simulink model "ejh61a"  (Simulink 3.00)
settings: Solver=ode45  StartTime=0.0  StopTime=10.0  RelTol=1e-3
values from neighbouring files (symbols this model uses):
  x = P_global(1,:)'    [contp5.m]    (also in ejh31.m = [0:0.2:5]; ejh62.m = 0:0.01:12; ejh63.m = 0:0.01:12)
  y = P_global(2,:)'    [contp5.m]    (also in ejh31.m = sqrt(25-x.^2); ejh62.m = 0:0.01:12; ejh63.m = 0:0.01:12)
undefined symbols (not defined in the file or in its folder): L
settings Model: LastModifiedBy=Administrador

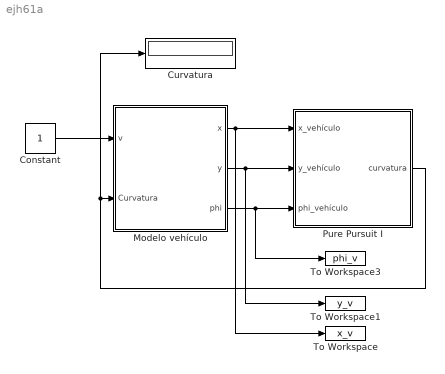
== system ejh61a ==
  Constant : Constant  Value=1
  Curvatura : Display
      settings: Format=short
  Modelo vehículo : Subsystem  mask{x_inicial=0, y_inicial=0.5, phi_inicial=0}
      mask prompts: x_inicial "Valor inicial de la coordenada x:"; y_inicial "Valor inicial de la coordenada y:"; phi_inicial "Valor inicial de la orientación:"
  Pure Pursuit I : Subsystem  mask(Pure Pursuit I){x_camino=x, y_camino=y, L=L}
      mask prompts: x_camino "Coordenadas x del camino:"; y_camino "Coordenadas y del camino:"; L "Parámetro Look-ahead (L):"
      mask help: Este bloque se encarga de calcular la curvatura que es necesario suministrar al vehículo cuando se emplea la técnica de persecución pura con el parámetro look-ahead (L) fijo.
      mask init:
      | global K_ANT
      | K_ANT=1;
  To Workspace : ToWorkspace  VariableName=x_v  SampleTime=-1  SaveFormat=Matrix
  To Workspace1 : ToWorkspace  VariableName=y_v  SampleTime=-1  SaveFormat=Matrix
  To Workspace3 : ToWorkspace  VariableName=phi_v  SampleTime=-1  SaveFormat=Matrix
  wires:
  Constant/1 -> Modelo vehículo/1(v)
  Modelo vehículo/1(x) -> To Workspace/1, Pure Pursuit I/1(x_vehículo)
  Pure Pursuit I/1(curvatura) -> Modelo vehículo/2(Curvatura), Curvatura/1
  Modelo vehículo/2(y) -> To Workspace1/1, Pure Pursuit I/2(y_vehículo)
  Modelo vehículo/3(phi) -> Pure Pursuit I/3(phi_vehículo), To Workspace3/1

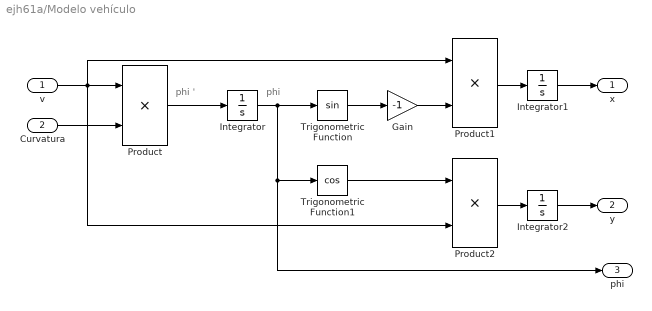
== system ejh61a/Modelo vehículo ==
  note: phi '
  note: phi
  v : Inport  Port=1  PortWidth=-1  SampleTime=-1  DataType=auto
      settings: SignalType=auto
  Curvatura : Inport  Port=2  PortWidth=-1  SampleTime=-1  DataType=auto
      settings: SignalType=auto
  Gain : Gain  Gain=-1  SaturateOnIntegerOverflow=on
  Integrator : Integrator  ExternalReset=none  InitialConditionSource=internal  InitialCondition=phi_inicial  LimitOutput=off  UpperSaturationLimit=inf  LowerSaturationLimit=-inf  ShowSaturationPort=off  ShowStatePort=off  AbsoluteTolerance=auto
  Integrator1 : Integrator  ExternalReset=none  InitialConditionSource=internal  InitialCondition=x_inicial  LimitOutput=off  UpperSaturationLimit=inf  LowerSaturationLimit=-inf  ShowSaturationPort=off  ShowStatePort=off  AbsoluteTolerance=auto
  Integrator2 : Integrator  ExternalReset=none  InitialConditionSource=internal  InitialCondition=y_inicial  LimitOutput=off  UpperSaturationLimit=inf  LowerSaturationLimit=-inf  ShowSaturationPort=off  ShowStatePort=off  AbsoluteTolerance=auto
  Product : Product  Inputs=2  SaturateOnIntegerOverflow=on
  Product1 : Product  Inputs=2  SaturateOnIntegerOverflow=on
  Product2 : Product  Inputs=2  SaturateOnIntegerOverflow=on
  Trigonometric Function : Trigonometry  Operator=sin  OutputSignalType=auto
  Trigonometric Function1 : Trigonometry  Operator=cos  OutputSignalType=auto
  x : Outport  Port=1
  y : Outport  Port=2
  phi : Outport  Port=3
  wires:
  Curvatura/1 -> Product/2
  Product/1 -> Integrator/1
  Integrator/1 -> Trigonometric Function/1, Trigonometric Function1/1, phi/1
  Trigonometric Function/1 -> Gain/1
  Gain/1 -> Product1/2
  v/1 -> Product/1, Product1/1, Product2/2
  Trigonometric Function1/1 -> Product2/1
  Product1/1 -> Integrator1/1
  Product2/1 -> Integrator2/1
  Integrator2/1 -> y/1
  Integrator1/1 -> x/1

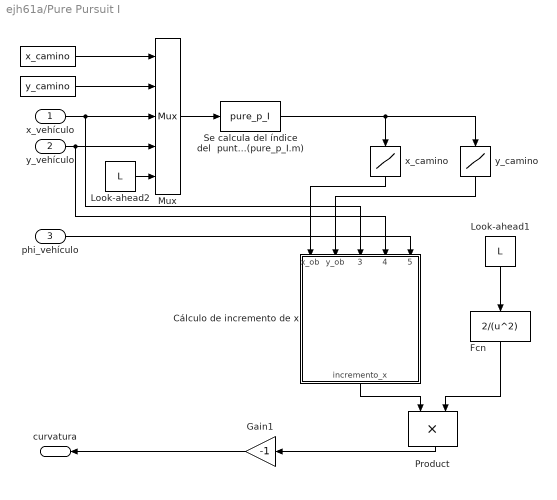
== system ejh61a/Pure Pursuit I ==
  x_vehículo : Inport  Port=1  PortWidth=-1  SampleTime=-1  DataType=auto
      settings: SignalType=auto
  y_vehículo : Inport  Port=2  PortWidth=-1  SampleTime=-1  DataType=auto
      settings: SignalType=auto
  phi_vehículo : Inport  Port=3  PortWidth=-1  SampleTime=-1  DataType=auto
      settings: SignalType=auto
  " " : Constant  Value=y_camino
  "  " : Constant  Value=x_camino
  Cálculo de incremento de x : Subsystem  Orientation=down
  Fcn : Fcn  Orientation=down  Expr=2/(u^2)
  Gain1 : Gain  Orientation=left  Gain=-1  SaturateOnIntegerOverflow=on
  Look-ahead1 : Constant  Orientation=down  Value=L
  Look-ahead2 : Constant  Value=L
  Mux : Mux  Inputs=5
      settings: DisplayOption=none
  Product : Product  Orientation=down  Inputs=2  SaturateOnIntegerOverflow=on
  Se calcula del índice del  punto que está a distancia L (pure_p_I.m) : MATLABFcn  MATLABFcn=pure_p_I  OutputWidth=-1  OutputSignalType=auto
  x_camino : Lookup  Orientation=down  InputValues=1:length(x_camino)  OutputValues=x_camino
  y_camino : Lookup  Orientation=down  InputValues=1:length(y_camino)  OutputValues=y_camino
  curvatura : Outport  Orientation=left  Port=1
  wires:
  Fcn/1 -> Product/2
  Look-ahead1/1 -> Fcn/1
  Se calcula del índice del  punto que está a distancia L (pure_p_I.m)/1 -> y_camino/1, x_camino/1
  y_camino/1 -> Cálculo de incremento de x/2(y_ob)
  x_camino/1 -> Cálculo de incremento de x/1(x_ob)
  Gain1/1 -> curvatura/1
  Product/1 -> Gain1/1
  "  "/1 -> Mux/1
  " "/1 -> Mux/2
  x_vehículo/1 -> Mux/3, Cálculo de incremento de x/3(x_vehículo)
  y_vehículo/1 -> Mux/4, Cálculo de incremento de x/4(y_vehículo)
  Look-ahead2/1 -> Mux/5
  Mux/1 -> Se calcula del índice del  punto que está a distancia L (pure_p_I.m)/1
  Cálculo de incremento de x/1(incremento_x) -> Product/1
  phi_vehículo/1 -> Cálculo de incremento de x/5(phi_vehículo)

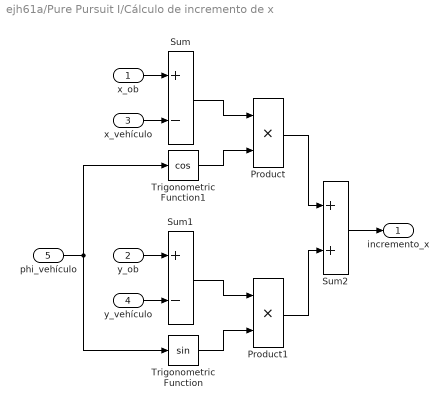
== system ejh61a/Pure Pursuit I/Cálculo de incremento de x ==
  x_ob : Inport  Port=1  PortWidth=-1  SampleTime=-1  DataType=auto
      settings: SignalType=auto
  y_ob : Inport  Port=2  PortWidth=-1  SampleTime=-1  DataType=auto
      settings: SignalType=auto
  x_vehículo : Inport  Port=3  PortWidth=-1  SampleTime=-1  DataType=auto
      settings: SignalType=auto
  y_vehículo : Inport  Port=4  PortWidth=-1  SampleTime=-1  DataType=auto
      settings: SignalType=auto
  phi_vehículo : Inport  Port=5  PortWidth=-1  SampleTime=-1  DataType=auto
      settings: SignalType=auto
  Product : Product  Inputs=2  SaturateOnIntegerOverflow=on
  Product1 : Product  Inputs=2  SaturateOnIntegerOverflow=on
  Sum : Sum  Inputs=+-  SaturateOnIntegerOverflow=on
  Sum1 : Sum  Inputs=+-  SaturateOnIntegerOverflow=on
  Sum2 : Sum  Inputs=++  SaturateOnIntegerOverflow=on
  Trigonometric Function : Trigonometry  Operator=sin  OutputSignalType=auto
  Trigonometric Function1 : Trigonometry  Operator=cos  OutputSignalType=auto
  incremento_x : Outport  Port=1
  wires:
  Sum2/1 -> incremento_x/1
  Product1/1 -> Sum2/2
  Product/1 -> Sum2/1
  Trigonometric Function/1 -> Product1/2
  Sum1/1 -> Product1/1
  phi_vehículo/1 -> Trigonometric Function/1, Trigonometric Function1/1
  Trigonometric Function1/1 -> Product/2
  Sum/1 -> Product/1
  y_vehículo/1 -> Sum1/2
  y_ob/1 -> Sum1/1
  x_vehículo/1 -> Sum/2
  x_ob/1 -> Sum/1
